simulink library "Massflow_Sensor"  (Simulink 8.2)
settings: Solver=ode45  StartTime=0.0  StopTime=10.0  RelTol=1e-3
settings Model: Creator=lena.frank  LastModifiedBy=drhf

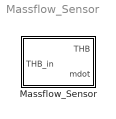
== system Massflow_Sensor ==
  Massflow_Sensor : Subsystem  mask(temperature measurement sensor){tc=10, t0=0}
      mask prompts: tc "time constant of sensor [s]"; t0 "initial value [kg/s]"
      mask help: Measurement sensor for temperatures with first-oder hold. Temperature is in degree centigrade.
      mask init:
      | tc = 1/max(tc, 0.001);
      mask Help: web(fullfile(path_carnot('help'),'Massflow_Sensor.html'),'-helpbrowser')

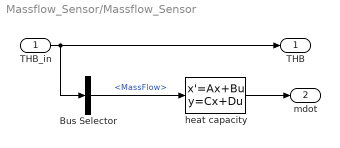
== system Massflow_Sensor/Massflow_Sensor ==
  THB_in : Inport
  Bus Selector : BusSelector  OutputSignals=MassFlow
  heat capacity : StateSpace  A=-tc  B=tc  D=0  X0=t0
  THB : Outport
  mdot : Outport  Port=2
  wires:
  heat capacity/1 -> mdot/1
  Bus Selector/1 -> heat capacity/1  "<MassFlow>"
  THB_in/1 -> Bus Selector/1, THB/1
